simulink model "mrefrobotarm_modified_previous_y_previous_u_previous_ref_pert_2"  (R2018b)
settings: Solver=FixedStepAuto  StartTime=0.0  StopTime=60  RelTol=1e-3  AbsTol=1e-6
undefined symbols (not defined in the file or in its folder): cc, options
libraries: neural x858, simulink x1
(part 8 of 32)

== system mrefrobotarm_modified_previous_y_previous_u_previous_ref_pert_2/m=0 sd=0 new/Layer 3/Delays 1 ==
  "p{3}" : Inport  PortDimensions=30
      mask Display: e = 0.06;c1 = [120 230 180]/255;c2 = ([120 230 180]+0)/(256+128);c3 = ([120 230 180]+128)/(256+128);patch([0 1 1 0],[0 0 1 1],c1);patch([0 1 1 1-e 1-e 0+e],[0 0 1 1-e 0+e 0+e],c2);patch([0 0 1 1-e 0+e 0+e],[0 1 1 1-e 1-e 0+e],c3);plot([0 1 1 0 0],[0 0 1 1 0]);
  mux : Mux  Inputs=1
      mask Display: e = 0.06;c1 = [120 150 230]/255;c2 = ([120 150 230]+0)/383;c3 = ([120 150 230]+128)/383;patch([0 1 1 0],[0 0 1 1],c1);patch([0 1 1 1-e 1-e 0+e],[0 0 1 1-e 0+e 0+e],c2);patch([0 0 1 1-e 0+e 0+e],[0 1 1 1-e 1-e 0+e],c3);plot([0 1 1 0 0],[0 0 1 1 0]);disp('Mux')
  "pd{3,2}" : Outport
      mask Display: e = 0.06;c1 = [120 230 180]/255;c2 = ([120 230 180]+0)/(256+128);c3 = ([120 230 180]+128)/(256+128);patch([0 1 1 0],[0 0 1 1],c1);patch([0 1 1 1-e 1-e 0+e],[0 0 1 1-e 0+e 0+e],c2);patch([0 0 1 1-e 0+e 0+e],[0 1 1 1-e 1-e 0+e],c3);plot([0 1 1 0 0],[0 0 1 1 0]);
  wires:
  "p{3}"/1 -> mux/1
  mux/1 -> "pd{3,2}"/1

== system mrefrobotarm_modified_previous_y_previous_u_previous_ref_pert_2/m=0 sd=0 new/Layer 3/LW{3,2} ==
  "ad{3,2}" : Inport  PortDimensions=30
      mask Display: e = 0.06;c1 = [120 230 180]/255;c2 = ([120 230 180]+0)/(256+128);c3 = ([120 230 180]+128)/(256+128);patch([0 1 1 0],[0 0 1 1],c1);patch([0 1 1 1-e 1-e 0+e],[0 0 1 1-e 0+e 0+e],c2);patch([0 0 1 1-e 0+e 0+e],[0 1 1 1-e 1-e 0+e],c3);plot([0 1 1 0 0],[0 0 1 1 0]);
  "IW{3,2}(1,:)'" : Constant  Value=[-0.131328794563046191701261022899416275322437286376953125;-0.2584338741751863732787342087249271571636199951171875;-0.0903219952940264858565200256634852848947048187255859375;-0.024805674677310464437685055827387259341776371002197265625;0.3313165319494135729883055319078266620635986328125;-0.1756848520066605912059998217955580912530422210693359375;0.62966251824317842622491525617078877985477447509765625;0.002210739002808526608434558369253863929770886898040771484375;0.003937183106850739543192130298621123074553906917572021484375;-0.0763844646287754613922516000457108020782470703125;0.08029708353647936613928237647996866144239902496337890625;-0.059445415608557324038674352095767972059547901153564453125;-0.4850157429702022238160452616284601390361785888671875;-0.1966069396515301159755750859403633512556552886962890625;0.015572684574274832380869071357665234245359897613525390625;0.10249042766198744602856862684348016045987606048583984375;0.259898651756895804343372446965076960623264312744140625;-0.007831826389256744958000666656516841612756252288818359375;-0.060342808177259003865611219907805207185447216033935546875;0.2102990586238534242990994016508921049535274505615234375;-0.054344878005701487133638494242404703982174396514892578125;-0.491551020946996597427158803839120082557201385498046875;-0.57063893253863418042470811997191049158573150634765625;-0.040752953733789419599187198173240176402032375335693359375;0.385146883729147571084894252635422162711620330810546875;-0.49669180336826268540306728027644567191600799560546875;-0.000294463483847452571484648586874754983000457286834716796875;0.402555479876675115225026502230321057140827178955078125;0.0840813874034800623480379044849541969597339630126953125;0.489528113088271099595516488989233039319515228271484375]
      mask Display: e = 0.06;c1 = [120 150 230]/255;c2 = ([120 150 230]+0)/383;c3 = ([120 150 230]+128)/383;patch([0 1 1 0],[0 0 1 1],c1);patch([0 1 1 1-e 1-e 0+e],[0 0 1 1-e 0+e 0+e],c2);patch([0 0 1 1-e 0+e 0+e],[0 1 1 1-e 1-e 0+e],c3);plot([0 1 1 0 0],[0 0 1 1 0]);disp('weights');
  Mux : Mux  Inputs=1
      mask Display: e = 0.06;c1 = [120 150 230]/255;c2 = ([120 150 230]+0)/383;c3 = ([120 150 230]+128)/383;patch([0 1 1 0],[0 0 1 1],c1);patch([0 1 1 1-e 1-e 0+e],[0 0 1 1-e 0+e 0+e],c2);patch([0 0 1 1-e 0+e 0+e],[0 1 1 1-e 1-e 0+e],c3);plot([0 1 1 0 0],[0 0 1 1 0]);disp('Mux');
  dotprod1 : neural/Weight Functions/dotprod
  "lz{3,2}" : Outport
      mask Display: e = 0.06;c1 = [120 230 180]/255;c2 = ([120 230 180]+0)/(256+128);c3 = ([120 230 180]+128)/(256+128);patch([0 1 1 0],[0 0 1 1],c1);patch([0 1 1 1-e 1-e 0+e],[0 0 1 1-e 0+e 0+e],c2);patch([0 0 1 1-e 0+e 0+e],[0 1 1 1-e 1-e 0+e],c3);plot([0 1 1 0 0],[0 0 1 1 0]);
  wires:
  "IW{3,2}(1,:)'"/1 -> dotprod1/1
  "ad{3,2}"/1 -> dotprod1/2
  dotprod1/1 -> Mux/1
  Mux/1 -> "lz{3,2}"/1

== system mrefrobotarm_modified_previous_y_previous_u_previous_ref_pert_2/m=0 sd=0 original/Layer 1/Delays 1 ==
  "p{1}" : Inport  PortDimensions=10
      mask Display: e = 0.06;c1 = [120 230 180]/255;c2 = ([120 230 180]+0)/(256+128);c3 = ([120 230 180]+128)/(256+128);patch([0 1 1 0],[0 0 1 1],c1);patch([0 1 1 1-e 1-e 0+e],[0 0 1 1-e 0+e 0+e],c2);patch([0 0 1 1-e 0+e 0+e],[0 1 1 1-e 1-e 0+e],c3);plot([0 1 1 0 0],[0 0 1 1 0]);
  mux : Mux  Inputs=1
      mask Display: e = 0.06;c1 = [120 150 230]/255;c2 = ([120 150 230]+0)/383;c3 = ([120 150 230]+128)/383;patch([0 1 1 0],[0 0 1 1],c1);patch([0 1 1 1-e 1-e 0+e],[0 0 1 1-e 0+e 0+e],c2);patch([0 0 1 1-e 0+e 0+e],[0 1 1 1-e 1-e 0+e],c3);plot([0 1 1 0 0],[0 0 1 1 0]);disp('Mux')
  "pd{1,1}" : Outport
      mask Display: e = 0.06;c1 = [120 230 180]/255;c2 = ([120 230 180]+0)/(256+128);c3 = ([120 230 180]+128)/(256+128);patch([0 1 1 0],[0 0 1 1],c1);patch([0 1 1 1-e 1-e 0+e],[0 0 1 1-e 0+e 0+e],c2);patch([0 0 1 1-e 0+e 0+e],[0 1 1 1-e 1-e 0+e],c3);plot([0 1 1 0 0],[0 0 1 1 0]);
  wires:
  "p{1}"/1 -> mux/1
  mux/1 -> "pd{1,1}"/1

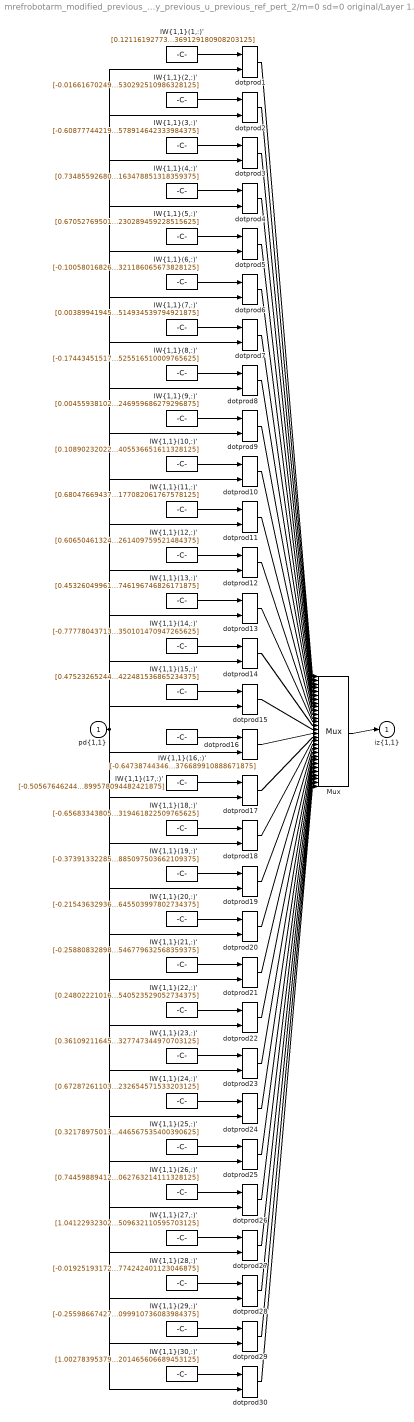
== system mrefrobotarm_modified_previous_y_previous_u_previous_ref_pert_2/m=0 sd=0 original/Layer 1/IW{1,1} ==
  "pd{1,1}" : Inport  PortDimensions=10
      mask Display: e = 0.06;c1 = [120 230 180]/255;c2 = ([120 230 180]+0)/(256+128);c3 = ([120 230 180]+128)/(256+128);patch([0 1 1 0],[0 0 1 1],c1);patch([0 1 1 1-e 1-e 0+e],[0 0 1 1-e 0+e 0+e],c2);patch([0 0 1 1-e 0+e 0+e],[0 1 1 1-e 1-e 0+e],c3);plot([0 1 1 0 0],[0 0 1 1 0]);
  "IW{1,1}(1,:)'" : Constant  Value=[0.12116192773643101598946003605306032113730907440185546875;-0.61504051461735576022960003683692775666713714599609375;0.1409010722643941893039709611912257969379425048828125;0.6780888328524288244381068579968996345996856689453125;1.099852074699011250658031713101081550121307373046875;0.1056636417972652564056801338665536604821681976318359375;-0.12249335544031504652284780831905663944780826568603515625;-1.023192361940513439577671306324191391468048095703125;0.52555112062766362601706759960507042706012725830078125;0.10235940031612085487910945857947808690369129180908203125]
      mask Display: e = 0.06;c1 = [120 150 230]/255;c2 = ([120 150 230]+0)/383;c3 = ([120 150 230]+128)/383;patch([0 1 1 0],[0 0 1 1],c1);patch([0 1 1 1-e 1-e 0+e],[0 0 1 1-e 0+e 0+e],c2);patch([0 0 1 1-e 0+e 0+e],[0 1 1 1-e 1-e 0+e],c3);plot([0 1 1 0 0],[0 0 1 1 0]);disp('Weights');
  "IW{1,1}(10,:)'" : Constant  Value=[0.10890232022583896942524717132982914336025714874267578125;0.65770880199305470359405489944037981331348419189453125;0.457449558769818132031304003248806111514568328857421875;0.78591806431375488273260998539626598358154296875;-0.2188123800257306961203340733845834620296955108642578125;-0.48560017494878715549333492162986658513545989990234375;0.69434633131231038305486436001956462860107421875;-0.328009816819692989753320944146253168582916259765625;0.476343472120701771910233901508036069571971893310546875;0.4472870790745435698454457451589405536651611328125]
      mask Display: e = 0.06;c1 = [120 150 230]/255;c2 = ([120 150 230]+0)/383;c3 = ([120 150 230]+128)/383;patch([0 1 1 0],[0 0 1 1],c1);patch([0 1 1 1-e 1-e 0+e],[0 0 1 1-e 0+e 0+e],c2);patch([0 0 1 1-e 0+e 0+e],[0 1 1 1-e 1-e 0+e],c3);plot([0 1 1 0 0],[0 0 1 1 0]);disp('Weights');
  "IW{1,1}(11,:)'" : Constant  Value=[0.680476694371919155202022011508233845233917236328125;-0.218609157014526156448397387066506780683994293212890625;0.6994701698477083784410979205858893692493438720703125;-0.75912984076269884869958559647784568369388580322265625;-0.053406333734809241509111643608775921165943145751953125;0.5067473596839289218252133650821633636951446533203125;-0.7233312131331359751129639334976673126220703125;0.0220245977869557851835935480266925878822803497314453125;-0.317828864736112548516899778405786491930484771728515625;-0.83728896145760878244601599362795241177082061767578125]
      mask Display: e = 0.06;c1 = [120 150 230]/255;c2 = ([120 150 230]+0)/383;c3 = ([120 150 230]+128)/383;patch([0 1 1 0],[0 0 1 1],c1);patch([0 1 1 1-e 1-e 0+e],[0 0 1 1-e 0+e 0+e],c2);patch([0 0 1 1-e 0+e 0+e],[0 1 1 1-e 1-e 0+e],c3);plot([0 1 1 0 0],[0 0 1 1 0]);disp('Weights');
  "IW{1,1}(12,:)'" : Constant  Value=[0.60650461324363258430736323134624399244785308837890625;0.48153819852384860400462684992817230522632598876953125;-0.04870024737972040995703792987114866264164447784423828125;-0.460239770351729193809120488367625512182712554931640625;-0.368942033692632731511906740706763230264186859130859375;-0.46185690513962518455315375831560231745243072509765625;0.72748634836911574286233417296898551285266876220703125;-0.1586777055629144117521178714014240540564060211181640625;-0.950068089025934536806516916840337216854095458984375;-1.257733091633853828028577481745742261409759521484375]
      mask Display: e = 0.06;c1 = [120 150 230]/255;c2 = ([120 150 230]+0)/383;c3 = ([120 150 230]+128)/383;patch([0 1 1 0],[0 0 1 1],c1);patch([0 1 1 1-e 1-e 0+e],[0 0 1 1-e 0+e 0+e],c2);patch([0 0 1 1-e 0+e 0+e],[0 1 1 1-e 1-e 0+e],c3);plot([0 1 1 0 0],[0 0 1 1 0]);disp('Weights');
  "IW{1,1}(13,:)'" : Constant  Value=[0.4532604996160010113470661963219754397869110107421875;0.09983497416402796476031511474502622149884700775146484375;0.3006063337801030410645353185827843844890594482421875;-0.09180389202883994237414100325622712261974811553955078125;-0.79528576080610113852031872738734818994998931884765625;-0.8960113888966159123583565815351903438568115234375;0.6124459313106982438768000065465457737445831298828125;-0.403120513671325564342140523876878432929515838623046875;0.275852681892310103162202494786470197141170501708984375;-0.9322307026330818313653026052634231746196746826171875]
      mask Display: e = 0.06;c1 = [120 150 230]/255;c2 = ([120 150 230]+0)/383;c3 = ([120 150 230]+128)/383;patch([0 1 1 0],[0 0 1 1],c1);patch([0 1 1 1-e 1-e 0+e],[0 0 1 1-e 0+e 0+e],c2);patch([0 0 1 1-e 0+e 0+e],[0 1 1 1-e 1-e 0+e],c3);plot([0 1 1 0 0],[0 0 1 1 0]);disp('Weights');
  "IW{1,1}(14,:)'" : Constant  Value=[-0.777780437137306268624570293468423187732696533203125;0.54311407500627495448242143538664095103740692138671875;0.1282828683578548789601114776814938522875308990478515625;-0.492876417301822022931645506105269305408000946044921875;0.16977207513145187167680205675424076616764068603515625;0.0156211573477218201855265533595229499042034149169921875;-0.446744619223521599593595965416170656681060791015625;0.75446679844643182999419650514028035104274749755859375;-0.92919935058635305669128001682111062109470367431640625;-0.77293975111376289621745172553346492350101470947265625]
      mask Display: e = 0.06;c1 = [120 150 230]/255;c2 = ([120 150 230]+0)/383;c3 = ([120 150 230]+128)/383;patch([0 1 1 0],[0 0 1 1],c1);patch([0 1 1 1-e 1-e 0+e],[0 0 1 1-e 0+e 0+e],c2);patch([0 0 1 1-e 0+e 0+e],[0 1 1 1-e 1-e 0+e],c3);plot([0 1 1 0 0],[0 0 1 1 0]);disp('Weights');
  "IW{1,1}(15,:)'" : Constant  Value=[0.475232652444419423343191510866745375096797943115234375;-0.96121566108966671748703447519801557064056396484375;-0.57026523941225215619255095589323900640010833740234375;0.377850789131591924263631199210067279636859893798828125;-0.246530389897684221178764119031256996095180511474609375;-0.2456529829883446203186991851907805539667606353759765625;-0.01169546179904616851896737017568739247508347034454345703125;0.04941958440568117172375650625326670706272125244140625;0.2692933235009551395933158346451818943023681640625;-0.98507416687839943758575600440963171422481536865234375]
      mask Display: e = 0.06;c1 = [120 150 230]/255;c2 = ([120 150 230]+0)/383;c3 = ([120 150 230]+128)/383;patch([0 1 1 0],[0 0 1 1],c1);patch([0 1 1 1-e 1-e 0+e],[0 0 1 1-e 0+e 0+e],c2);patch([0 0 1 1-e 0+e 0+e],[0 1 1 1-e 1-e 0+e],c3);plot([0 1 1 0 0],[0 0 1 1 0]);disp('Weights');
  "IW{1,1}(16,:)'" : Constant  Value=[-0.6473874434633859475951567219453863799571990966796875;0.07619240517464466455610505590811953879892826080322265625;0.60985403944523730590532295536831952631473541259765625;0.4716409511471406634797176593565382063388824462890625;-0.9407261485054314587017643134458921849727630615234375;0.469394008329378664701181378404726274311542510986328125;0.86159731456515220582303982155281119048595428466796875;-0.264297224920746531839910176131525076925754547119140625;0.378541128305662055719693626087973825633525848388671875;0.0612841587337953352943031859467737376689910888671875]
      mask Display: e = 0.06;c1 = [120 150 230]/255;c2 = ([120 150 230]+0)/383;c3 = ([120 150 230]+128)/383;patch([0 1 1 0],[0 0 1 1],c1);patch([0 1 1 1-e 1-e 0+e],[0 0 1 1-e 0+e 0+e],c2);patch([0 0 1 1-e 0+e 0+e],[0 1 1 1-e 1-e 0+e],c3);plot([0 1 1 0 0],[0 0 1 1 0]);disp('Weights');
  "IW{1,1}(17,:)'" : Constant  Value=[-0.50567646244606390126818951102904975414276123046875;-0.58678927891174470499180415572482161223888397216796875;-0.74791607997321796208467503674910403788089752197265625;0.09226660376835309207432800349124590866267681121826171875;-0.92881420303231576607316810623160563409328460693359375;0.2054439465067338377313177488758810795843601226806640625;-0.06644508752851059629751517832119134254753589630126953125;-0.0218069911409425921944293946808102191425859928131103515625;-0.4008602233399602976504638718324713408946990966796875;-0.20735309908321475358405905353720299899578094482421875]
      mask Display: e = 0.06;c1 = [120 150 230]/255;c2 = ([120 150 230]+0)/383;c3 = ([120 150 230]+128)/383;patch([0 1 1 0],[0 0 1 1],c1);patch([0 1 1 1-e 1-e 0+e],[0 0 1 1-e 0+e 0+e],c2);patch([0 0 1 1-e 0+e 0+e],[0 1 1 1-e 1-e 0+e],c3);plot([0 1 1 0 0],[0 0 1 1 0]);disp('Weights');
  "IW{1,1}(18,:)'" : Constant  Value=[-0.65683343805488114686141898346249945461750030517578125;0.58491845632951022793122319853864610195159912109375;-0.59386776290678866541128400058369152247905731201171875;0.3328090742596827578125839863787405192852020263671875;-0.40228141483918589127455334164551459252834320068359375;0.56176553124188155496909757857793010771274566650390625;-0.2134990708425597294439768347729113884270191192626953125;0.179285623717090170092802736689918674528598785400390625;0.68978737180453542077174233781988732516765594482421875;0.08143197107304323001386592295602895319461822509765625]
      mask Display: e = 0.06;c1 = [120 150 230]/255;c2 = ([120 150 230]+0)/383;c3 = ([120 150 230]+128)/383;patch([0 1 1 0],[0 0 1 1],c1);patch([0 1 1 1-e 1-e 0+e],[0 0 1 1-e 0+e 0+e],c2);patch([0 0 1 1-e 0+e 0+e],[0 1 1 1-e 1-e 0+e],c3);plot([0 1 1 0 0],[0 0 1 1 0]);disp('Weights');
  "IW{1,1}(19,:)'" : Constant  Value=[-0.37391332285017286896078303470858372747898101806640625;-0.41655114369798862394844718437525443732738494873046875;-0.722962656029874750629460322670638561248779296875;0.74460868870904572958124845172278583049774169921875;0.12195982058353192767352624059640220366418361663818359375;0.573352625586788011702310541295446455478668212890625;-0.6910118607599298190535819230717606842517852783203125;-0.142900412155376133060968868448981083929538726806640625;0.359668576337890122385232416490907780826091766357421875;0.94236811046126600643901838338933885097503662109375]
      mask Display: e = 0.06;c1 = [120 150 230]/255;c2 = ([120 150 230]+0)/383;c3 = ([120 150 230]+128)/383;patch([0 1 1 0],[0 0 1 1],c1);patch([0 1 1 1-e 1-e 0+e],[0 0 1 1-e 0+e 0+e],c2);patch([0 0 1 1-e 0+e 0+e],[0 1 1 1-e 1-e 0+e],c3);plot([0 1 1 0 0],[0 0 1 1 0]);disp('Weights');
  "IW{1,1}(2,:)'" : Constant  Value=[-0.0166167024917292759089715303844059235416352748870849609375;-0.357126463452990094982197888384689576923847198486328125;-0.916084382600150348707757075317203998565673828125;0.48655534141628298261395002555218525230884552001953125;-0.6016239976947996836997845093719661235809326171875;0.2604062173688583836650423108949325978755950927734375;-0.76106782890995205992368255465407855808734893798828125;0.68944498864043690655734053507330827414989471435546875;-0.749670894554280042854088605963625013828277587890625;-0.50522142973601547044637527505983598530292510986328125]
      mask Display: e = 0.06;c1 = [120 150 230]/255;c2 = ([120 150 230]+0)/383;c3 = ([120 150 230]+128)/383;patch([0 1 1 0],[0 0 1 1],c1);patch([0 1 1 1-e 1-e 0+e],[0 0 1 1-e 0+e 0+e],c2);patch([0 0 1 1-e 0+e 0+e],[0 1 1 1-e 1-e 0+e],c3);plot([0 1 1 0 0],[0 0 1 1 0]);disp('Weights');
  "IW{1,1}(20,:)'" : Constant  Value=[-0.2154363293600259077198444401801680214703083038330078125;0.50329604582178533167535761094768531620502471923828125;0.2169027594365723066172080280011869035661220550537109375;-0.1924528806850759055091515392632572911679744720458984375;0.7673985167013552821657640379271470010280609130859375;-0.90934673281269251532421549200080335140228271484375;-0.0087332413715192173941925801727848011068999767303466796875;-0.06668438227395256934215694855083711445331573486328125;-0.016986997923331130511126474402772146277129650115966796875;-0.53458303631503178987571800462319515645503997802734375]
      mask Display: e = 0.06;c1 = [120 150 230]/255;c2 = ([120 150 230]+0)/383;c3 = ([120 150 230]+128)/383;patch([0 1 1 0],[0 0 1 1],c1);patch([0 1 1 1-e 1-e 0+e],[0 0 1 1-e 0+e 0+e],c2);patch([0 0 1 1-e 0+e 0+e],[0 1 1 1-e 1-e 0+e],c3);plot([0 1 1 0 0],[0 0 1 1 0]);disp('Weights');
  "IW{1,1}(21,:)'" : Constant  Value=[-0.258808328980351609605037310757325030863285064697265625;-0.45559647879383280422160851230728439986705780029296875;0.93620596257909582948997240237076766788959503173828125;-0.142913494694684839458886926877312362194061279296875;-0.6309221664067627965977180792833678424358367919921875;0.09462987497119475233109398004671675153076648712158203125;-0.196676609376249034166761475717066787183284759521484375;0.340897810232632381133299759312649257481098175048828125;-0.60326966103195489576904719797312282025814056396484375;-0.1614198301976775551391796170719317160546779632568359375]
      mask Display: e = 0.06;c1 = [120 150 230]/255;c2 = ([120 150 230]+0)/383;c3 = ([120 150 230]+128)/383;patch([0 1 1 0],[0 0 1 1],c1);patch([0 1 1 1-e 1-e 0+e],[0 0 1 1-e 0+e 0+e],c2);patch([0 0 1 1-e 0+e 0+e],[0 1 1 1-e 1-e 0+e],c3);plot([0 1 1 0 0],[0 0 1 1 0]);disp('Weights');
  "IW{1,1}(22,:)'" : Constant  Value=[0.2480222101606265050488531187511398456990718841552734375;0.09883537976841751115930634341566474176943302154541015625;-0.54001494512905789946444201632402837276458740234375;-0.526715938672090100425293712760321795940399169921875;0.58119636565368903990957960559171624481678009033203125;0.37277994148824034059686027831048704683780670166015625;0.5963367799875081143312627318664453923702239990234375;0.0065429653912110440072691375235081068240106105804443359375;-0.73075576347838533397549554138095118105411529541015625;0.6130343513817047007563587612821720540523529052734375]
      mask Display: e = 0.06;c1 = [120 150 230]/255;c2 = ([120 150 230]+0)/383;c3 = ([120 150 230]+128)/383;patch([0 1 1 0],[0 0 1 1],c1);patch([0 1 1 1-e 1-e 0+e],[0 0 1 1-e 0+e 0+e],c2);patch([0 0 1 1-e 0+e 0+e],[0 1 1 1-e 1-e 0+e],c3);plot([0 1 1 0 0],[0 0 1 1 0]);disp('Weights');
  "IW{1,1}(23,:)'" : Constant  Value=[0.36109211645897498765833688594284467399120330810546875;0.54290639213263347517823831367422826588153839111328125;0.07594005242914191045056071516228257678449153900146484375;-0.2461072773103850364062594735514721833169460296630859375;-0.83697661529656885992523029926815070211887359619140625;0.9408581410656988719409810073557309806346893310546875;-0.468248142498214947604395774760632775723934173583984375;-0.2143536848566931218851294715932453982532024383544921875;0.3274754933856305338935044346726499497890472412109375;-0.132677823786770343605923017094028182327747344970703125]
      mask Display: e = 0.06;c1 = [120 150 230]/255;c2 = ([120 150 230]+0)/383;c3 = ([120 150 230]+128)/383;patch([0 1 1 0],[0 0 1 1],c1);patch([0 1 1 1-e 1-e 0+e],[0 0 1 1-e 0+e 0+e],c2);patch([0 0 1 1-e 0+e 0+e],[0 1 1 1-e 1-e 0+e],c3);plot([0 1 1 0 0],[0 0 1 1 0]);disp('Weights');
  "IW{1,1}(24,:)'" : Constant  Value=[0.6728726110333596022172741868416778743267059326171875;-0.8539407689115485755593226713244803249835968017578125;0.58299054175247189135689040995202958583831787109375;0.5965624611944964073018127237446606159210205078125;0.6125643432399214827199784849653951823711395263671875;-0.63478040904533561405997943438705988228321075439453125;-0.32505227239285205964591796146123670041561126708984375;-0.333898527368930275738279078723280690610408782958984375;0.47305369145102804662172957250731997191905975341796875;-0.5194015100786106842178924125619232654571533203125]
      mask Display: e = 0.06;c1 = [120 150 230]/255;c2 = ([120 150 230]+0)/383;c3 = ([120 150 230]+128)/383;patch([0 1 1 0],[0 0 1 1],c1);patch([0 1 1 1-e 1-e 0+e],[0 0 1 1-e 0+e 0+e],c2);patch([0 0 1 1-e 0+e 0+e],[0 1 1 1-e 1-e 0+e],c3);plot([0 1 1 0 0],[0 0 1 1 0]);disp('Weights');
  "IW{1,1}(25,:)'" : Constant  Value=[0.321789750139932217987137619275017641484737396240234375;-0.91569031640294495932863583220751024782657623291015625;-0.333761809396514841363767800430650822818279266357421875;0.7720546237362537755899438707274384796619415283203125;0.51198543788465411541466210110229440033435821533203125;0.824723342100778467056443332694470882415771484375;-0.33046471004821231787218493991531431674957275390625;-0.389875021002500543598756621577194891870021820068359375;0.5404086892708424016973367542959749698638916015625;0.330923257377163049230972546865814365446567535400390625]
      mask Display: e = 0.06;c1 = [120 150 230]/255;c2 = ([120 150 230]+0)/383;c3 = ([120 150 230]+128)/383;patch([0 1 1 0],[0 0 1 1],c1);patch([0 1 1 1-e 1-e 0+e],[0 0 1 1-e 0+e 0+e],c2);patch([0 0 1 1-e 0+e 0+e],[0 1 1 1-e 1-e 0+e],c3);plot([0 1 1 0 0],[0 0 1 1 0]);disp('Weights');
  "IW{1,1}(26,:)'" : Constant  Value=[0.74459889412126256669210988548002205789089202880859375;-0.92984896899672364600775154030998237431049346923828125;0.37858439602939097934353185337386094033718109130859375;-0.198109382923818466704091179053648374974727630615234375;0.8930802272104247929718212617444805800914764404296875;-0.08305259436108174131430104125684010796248912811279296875;0.2584402796521445555555374085088260471820831298828125;-0.1276313566322919423878801126193138770759105682373046875;0.129711283535910160136239710482186637818813323974609375;0.8884779581083848132294633614947088062763214111328125]
      mask Display: e = 0.06;c1 = [120 150 230]/255;c2 = ([120 150 230]+0)/383;c3 = ([120 150 230]+128)/383;patch([0 1 1 0],[0 0 1 1],c1);patch([0 1 1 1-e 1-e 0+e],[0 0 1 1-e 0+e 0+e],c2);patch([0 0 1 1-e 0+e 0+e],[0 1 1 1-e 1-e 0+e],c3);plot([0 1 1 0 0],[0 0 1 1 0]);disp('Weights');
  "IW{1,1}(27,:)'" : Constant  Value=[1.0412293230277336331113247069879435002803802490234375;0.378240268704322979420595629562740214169025421142578125;0.07225563123705869283952551995753310620784759521484375;-0.84672746672924736888177221771911717951297760009765625;-0.92490468420280269601363443143782205879688262939453125;0.22823534262087463719836932796170003712177276611328125;-0.73329745087433939598753340760595165193080902099609375;0.1683653579491500018594507537272875197231769561767578125;-0.017424600058409463188002774813867290504276752471923828125;-0.341270477338222744112528062032652087509632110595703125]
      mask Display: e = 0.06;c1 = [120 150 230]/255;c2 = ([120 150 230]+0)/383;c3 = ([120 150 230]+128)/383;patch([0 1 1 0],[0 0 1 1],c1);patch([0 1 1 1-e 1-e 0+e],[0 0 1 1-e 0+e 0+e],c2);patch([0 0 1 1-e 0+e 0+e],[0 1 1 1-e 1-e 0+e],c3);plot([0 1 1 0 0],[0 0 1 1 0]);disp('Weights');
  "IW{1,1}(28,:)'" : Constant  Value=[-0.019251931722092309462457393465228960849344730377197265625;0.335699510860663907774181780041544698178768157958984375;-0.22472946705043839177307063437183387577533721923828125;0.315214660686319703142288517483393661677837371826171875;-0.176498236704149602527280649155727587640285491943359375;0.31912578476095332380424451912404038012027740478515625;1.1358118760290063509188485113554634153842926025390625;0.50415117773524731337175808221218176186084747314453125;0.2886850425787861329496308826492168009281158447265625;0.7670891568288478179482581253978423774242401123046875]
      mask Display: e = 0.06;c1 = [120 150 230]/255;c2 = ([120 150 230]+0)/383;c3 = ([120 150 230]+128)/383;patch([0 1 1 0],[0 0 1 1],c1);patch([0 1 1 1-e 1-e 0+e],[0 0 1 1-e 0+e 0+e],c2);patch([0 0 1 1-e 0+e 0+e],[0 1 1 1-e 1-e 0+e],c3);plot([0 1 1 0 0],[0 0 1 1 0]);disp('Weights');
  "IW{1,1}(29,:)'" : Constant  Value=[-0.2559866742778955650550187783665023744106292724609375;-0.71127991086725816938240996023523621261119842529296875;-0.41043610779858941128850347013212740421295166015625;0.7048722895097139229392269044183194637298583984375;-0.221963796580707306560498182079754769802093505859375;0.5617244972289625604133789238403551280498504638671875;-0.771930415379233014760984588065184652805328369140625;-0.78155030395383284780308486006106249988079071044921875;0.565621064146131669048145340639166533946990966796875;0.413091510285398921809019157080911099910736083984375]
      mask Display: e = 0.06;c1 = [120 150 230]/255;c2 = ([120 150 230]+0)/383;c3 = ([120 150 230]+128)/383;patch([0 1 1 0],[0 0 1 1],c1);patch([0 1 1 1-e 1-e 0+e],[0 0 1 1-e 0+e 0+e],c2);patch([0 0 1 1-e 0+e 0+e],[0 1 1 1-e 1-e 0+e],c3);plot([0 1 1 0 0],[0 0 1 1 0]);disp('Weights');
  "IW{1,1}(3,:)'" : Constant  Value=[-0.608777442190258977205985502223484218120574951171875;0.85799971456095480704107103520072996616363525390625;-0.74962009257192441236128388482029549777507781982421875;0.192139323756343849414207625159178860485553741455078125;-0.414085422551569493077039396666805259883403778076171875;-0.406854972792761060418342822231352329254150390625;0.484699008415858278997490060646669007837772369384765625;0.285487826019434287605491817885194905102252960205078125;0.56545161713676106440829016719362698495388031005859375;0.09239905289283210920725508685791282914578914642333984375]
      mask Display: e = 0.06;c1 = [120 150 230]/255;c2 = ([120 150 230]+0)/383;c3 = ([120 150 230]+128)/383;patch([0 1 1 0],[0 0 1 1],c1);patch([0 1 1 1-e 1-e 0+e],[0 0 1 1-e 0+e 0+e],c2);patch([0 0 1 1-e 0+e 0+e],[0 1 1 1-e 1-e 0+e],c3);plot([0 1 1 0 0],[0 0 1 1 0]);disp('Weights');
  "IW{1,1}(30,:)'" : Constant  Value=[1.0027839537988934015544373323791660368442535400390625;0.349433229052273919279514302616007626056671142578125;0.362556071783007194397896455484442412853240966796875;-0.250092465292030718959637169973575510084629058837890625;-0.69123761895338731164883938618004322052001953125;0.60623428321575023591805120304343290627002716064453125;-0.0997625681266436081795490053991670720279216766357421875;0.67615237979682085711630179503117688000202178955078125;0.271067671262654796837665571729303337633609771728515625;-0.00512115152377713885034626883907549199648201465606689453125]
      mask Display: e = 0.06;c1 = [120 150 230]/255;c2 = ([120 150 230]+0)/383;c3 = ([120 150 230]+128)/383;patch([0 1 1 0],[0 0 1 1],c1);patch([0 1 1 1-e 1-e 0+e],[0 0 1 1-e 0+e 0+e],c2);patch([0 0 1 1-e 0+e 0+e],[0 1 1 1-e 1-e 0+e],c3);plot([0 1 1 0 0],[0 0 1 1 0]);disp('Weights');
  "IW{1,1}(4,:)'" : Constant  Value=[0.734855926809820036993414760218001902103424072265625;-0.389570311948177872007903488338342867791652679443359375;-0.81885738937908192358605674598948098719120025634765625;1.0182410106540238370342876805807463824748992919921875;-0.464000445312876375059119027355336584150791168212890625;0.212478053400078359391756066543166525661945343017578125;-0.200652031357742732797788676180061884224414825439453125;-0.52859242807870743252607326212455518543720245361328125;-0.77201313289327100353176547287148423492908477783203125;-0.239873280292042689865184001973830163478851318359375]
      mask Display: e = 0.06;c1 = [120 150 230]/255;c2 = ([120 150 230]+0)/383;c3 = ([120 150 230]+128)/383;patch([0 1 1 0],[0 0 1 1],c1);patch([0 1 1 1-e 1-e 0+e],[0 0 1 1-e 0+e 0+e],c2);patch([0 0 1 1-e 0+e 0+e],[0 1 1 1-e 1-e 0+e],c3);plot([0 1 1 0 0],[0 0 1 1 0]);disp('Weights');
  "IW{1,1}(5,:)'" : Constant  Value=[0.67052769501434095200664842195692472159862518310546875;-0.2152872761339806040314925894563202746212482452392578125;0.384828281605536004494894086747081018984317779541015625;-0.6757215826549491932695445939316414296627044677734375;-0.327717615916509108497933766557252965867519378662109375;0.944927686673076028256446079467423260211944580078125;0.85313206769565919085351879402878694236278533935546875;0.26416739724157023427864032782963477075099945068359375;0.429525654215454466555712542685796506702899932861328125;0.1272253550685261969110939617166877724230289459228515625]
      mask Display: e = 0.06;c1 = [120 150 230]/255;c2 = ([120 150 230]+0)/383;c3 = ([120 150 230]+128)/383;patch([0 1 1 0],[0 0 1 1],c1);patch([0 1 1 1-e 1-e 0+e],[0 0 1 1-e 0+e 0+e],c2);patch([0 0 1 1-e 0+e 0+e],[0 1 1 1-e 1-e 0+e],c3);plot([0 1 1 0 0],[0 0 1 1 0]);disp('Weights');
  "IW{1,1}(6,:)'" : Constant  Value=[-0.100580168262270841506023089095833711326122283935546875;-0.82821855871360516854196021085954271256923675537109375;-0.8808772026876916516613391650025732815265655517578125;0.252657513681145307060660343267954885959625244140625;-0.2275202493627272726239851863283547572791576385498046875;0.0031599064136631741135652351459839337621815502643585205078125;-0.310595503818927198835808667354285717010498046875;0.26256673153875331738760223743156529963016510009765625;0.1747747259452554491332421093829907476902008056640625;1.07499825327508791161790213664062321186065673828125]
      mask Display: e = 0.06;c1 = [120 150 230]/255;c2 = ([120 150 230]+0)/383;c3 = ([120 150 230]+128)/383;patch([0 1 1 0],[0 0 1 1],c1);patch([0 1 1 1-e 1-e 0+e],[0 0 1 1-e 0+e 0+e],c2);patch([0 0 1 1-e 0+e 0+e],[0 1 1 1-e 1-e 0+e],c3);plot([0 1 1 0 0],[0 0 1 1 0]);disp('Weights');
  "IW{1,1}(7,:)'" : Constant  Value=[0.0038994194597327630318062130498901751707307994365692138671875;0.67040660914633110056826126310625113546848297119140625;-0.6677336897836270157569060756941325962543487548828125;0.681750229707159149938888731412589550018310546875;-0.485568612997461845903757193809724412858486175537109375;0.36692165947515043011861735067213885486125946044921875;0.72294597873417465461187703112955205142498016357421875;0.540634884828998796280075112008489668369293212890625;-0.434902593385109559331880291210836730897426605224609375;0.6714108410792796188815145796979777514934539794921875]
      mask Display: e = 0.06;c1 = [120 150 230]/255;c2 = ([120 150 230]+0)/383;c3 = ([120 150 230]+128)/383;patch([0 1 1 0],[0 0 1 1],c1);patch([0 1 1 1-e 1-e 0+e],[0 0 1 1-e 0+e 0+e],c2);patch([0 0 1 1-e 0+e 0+e],[0 1 1 1-e 1-e 0+e],c3);plot([0 1 1 0 0],[0 0 1 1 0]);disp('Weights');
  "IW{1,1}(8,:)'" : Constant  Value=[-0.1744345151722600240074001476386911235749721527099609375;-0.368943390105170021531222346311551518738269805908203125;-0.4749454777973067809426765961688943207263946533203125;-0.247239983075249802890738237692858092486858367919921875;0.44350679069850296176724668839597143232822418212890625;0.0102347645488580739348005721467416151426732540130615234375;-0.6757733816479476463001674346742220222949981689453125;0.1963547136057247899376676514293649233877658843994140625;-0.90150897032444399226136511060758493840694427490234375;0.7111578829426312697847833987907506525516510009765625]
      mask Display: e = 0.06;c1 = [120 150 230]/255;c2 = ([120 150 230]+0)/383;c3 = ([120 150 230]+128)/383;patch([0 1 1 0],[0 0 1 1],c1);patch([0 1 1 1-e 1-e 0+e],[0 0 1 1-e 0+e 0+e],c2);patch([0 0 1 1-e 0+e 0+e],[0 1 1 1-e 1-e 0+e],c3);plot([0 1 1 0 0],[0 0 1 1 0]);disp('Weights');
  "IW{1,1}(9,:)'" : Constant  Value=[0.00455938102191570139576359821376172476448118686676025390625;-0.31708861445531477674109055442386306822299957275390625;-0.5208088157022745523505591336288489401340484619140625;-0.2438961511069205612134425109616131521761417388916015625;-0.63715103832776998071807383894338272511959075927734375;-0.745227629189292972711200491175986826419830322265625;-0.591068850718129201737838229746557772159576416015625;0.69980425656285538682510605212883092463016510009765625;0.392129580075222694546255297609604895114898681640625;0.69171599388173188316386585938744246959686279296875]
      mask Display: e = 0.06;c1 = [120 150 230]/255;c2 = ([120 150 230]+0)/383;c3 = ([120 150 230]+128)/383;patch([0 1 1 0],[0 0 1 1],c1);patch([0 1 1 1-e 1-e 0+e],[0 0 1 1-e 0+e 0+e],c2);patch([0 0 1 1-e 0+e 0+e],[0 1 1 1-e 1-e 0+e],c3);plot([0 1 1 0 0],[0 0 1 1 0]);disp('Weights');
  Mux : Mux  Inputs=30
      mask Display: e = 0.06;c1 = [120 150 230]/255;c2 = ([120 150 230]+0)/383;c3 = ([120 150 230]+128)/383;patch([0 1 1 0],[0 0 1 1],c1);patch([0 1 1 1-e 1-e 0+e],[0 0 1 1-e 0+e 0+e],c2);patch([0 0 1 1-e 0+e 0+e],[0 1 1 1-e 1-e 0+e],c3);plot([0 1 1 0 0],[0 0 1 1 0]);disp('Mux');
  dotprod{1..30} (30 alike) : neural/Weight Functions/dotprod
  "iz{1,1}" : Outport
      mask Display: e = 0.06;c1 = [120 230 180]/255;c2 = ([120 230 180]+0)/(256+128);c3 = ([120 230 180]+128)/(256+128);patch([0 1 1 0],[0 0 1 1],c1);patch([0 1 1 1-e 1-e 0+e],[0 0 1 1-e 0+e 0+e],c2);patch([0 0 1 1-e 0+e 0+e],[0 1 1 1-e 1-e 0+e],c3);plot([0 1 1 0 0],[0 0 1 1 0]);
  wires:
  "IW{1,1}(1,:)'"/1 -> dotprod1/1
  "pd{1,1}"/1 -> dotprod1/2, dotprod2/2, dotprod3/2, dotprod4/2, dotprod5/2, dotprod6/2, dotprod7/2, dotprod8/2, dotprod9/2, dotprod10/2, dotprod11/2, dotprod12/2, dotprod13/2, dotprod14/2, dotprod15/2, dotprod16/2, dotprod17/2, dotprod18/2, dotprod19/2, dotprod20/2, dotprod21/2, dotprod22/2, dotprod23/2, dotprod24/2, dotprod25/2, dotprod26/2, dotprod27/2, dotprod28/2, dotprod29/2, dotprod30/2
  dotprod1/1 -> Mux/1
  "IW{1,1}(2,:)'"/1 -> dotprod2/1
  dotprod2/1 -> Mux/2
  "IW{1,1}(3,:)'"/1 -> dotprod3/1
  dotprod3/1 -> Mux/3
  "IW{1,1}(4,:)'"/1 -> dotprod4/1
  dotprod4/1 -> Mux/4
  "IW{1,1}(5,:)'"/1 -> dotprod5/1
  dotprod5/1 -> Mux/5
  "IW{1,1}(6,:)'"/1 -> dotprod6/1
  dotprod6/1 -> Mux/6
  "IW{1,1}(7,:)'"/1 -> dotprod7/1
  dotprod7/1 -> Mux/7
  "IW{1,1}(8,:)'"/1 -> dotprod8/1
  dotprod8/1 -> Mux/8
  "IW{1,1}(9,:)'"/1 -> dotprod9/1
  dotprod9/1 -> Mux/9
  "IW{1,1}(10,:)'"/1 -> dotprod10/1
  dotprod10/1 -> Mux/10
  "IW{1,1}(11,:)'"/1 -> dotprod11/1
  dotprod11/1 -> Mux/11
  "IW{1,1}(12,:)'"/1 -> dotprod12/1
  dotprod12/1 -> Mux/12
  "IW{1,1}(13,:)'"/1 -> dotprod13/1
  dotprod13/1 -> Mux/13
  "IW{1,1}(14,:)'"/1 -> dotprod14/1
  dotprod14/1 -> Mux/14
  "IW{1,1}(15,:)'"/1 -> dotprod15/1
  dotprod15/1 -> Mux/15
  "IW{1,1}(16,:)'"/1 -> dotprod16/1
  dotprod16/1 -> Mux/16
  "IW{1,1}(17,:)'"/1 -> dotprod17/1
  dotprod17/1 -> Mux/17
  "IW{1,1}(18,:)'"/1 -> dotprod18/1
  dotprod18/1 -> Mux/18
  "IW{1,1}(19,:)'"/1 -> dotprod19/1
  dotprod19/1 -> Mux/19
  "IW{1,1}(20,:)'"/1 -> dotprod20/1
  dotprod20/1 -> Mux/20
  "IW{1,1}(21,:)'"/1 -> dotprod21/1
  dotprod21/1 -> Mux/21
  "IW{1,1}(22,:)'"/1 -> dotprod22/1
  dotprod22/1 -> Mux/22
  "IW{1,1}(23,:)'"/1 -> dotprod23/1
  dotprod23/1 -> Mux/23
  "IW{1,1}(24,:)'"/1 -> dotprod24/1
  dotprod24/1 -> Mux/24
  "IW{1,1}(25,:)'"/1 -> dotprod25/1
  dotprod25/1 -> Mux/25
  "IW{1,1}(26,:)'"/1 -> dotprod26/1
  dotprod26/1 -> Mux/26
  "IW{1,1}(27,:)'"/1 -> dotprod27/1
  dotprod27/1 -> Mux/27
  "IW{1,1}(28,:)'"/1 -> dotprod28/1
  dotprod28/1 -> Mux/28
  "IW{1,1}(29,:)'"/1 -> dotprod29/1
  dotprod29/1 -> Mux/29
  "IW{1,1}(30,:)'"/1 -> dotprod30/1
  dotprod30/1 -> Mux/30
  Mux/1 -> "iz{1,1}"/1

== system mrefrobotarm_modified_previous_y_previous_u_previous_ref_pert_2/m=0 sd=0 original/Layer 2/Delays 1 ==
  "p{2}" : Inport  PortDimensions=30
      mask Display: e = 0.06;c1 = [120 230 180]/255;c2 = ([120 230 180]+0)/(256+128);c3 = ([120 230 180]+128)/(256+128);patch([0 1 1 0],[0 0 1 1],c1);patch([0 1 1 1-e 1-e 0+e],[0 0 1 1-e 0+e 0+e],c2);patch([0 0 1 1-e 0+e 0+e],[0 1 1 1-e 1-e 0+e],c3);plot([0 1 1 0 0],[0 0 1 1 0]);
  mux : Mux  Inputs=1
      mask Display: e = 0.06;c1 = [120 150 230]/255;c2 = ([120 150 230]+0)/383;c3 = ([120 150 230]+128)/383;patch([0 1 1 0],[0 0 1 1],c1);patch([0 1 1 1-e 1-e 0+e],[0 0 1 1-e 0+e 0+e],c2);patch([0 0 1 1-e 0+e 0+e],[0 1 1 1-e 1-e 0+e],c3);plot([0 1 1 0 0],[0 0 1 1 0]);disp('Mux')
  "pd{2,1}" : Outport
      mask Display: e = 0.06;c1 = [120 230 180]/255;c2 = ([120 230 180]+0)/(256+128);c3 = ([120 230 180]+128)/(256+128);patch([0 1 1 0],[0 0 1 1],c1);patch([0 1 1 1-e 1-e 0+e],[0 0 1 1-e 0+e 0+e],c2);patch([0 0 1 1-e 0+e 0+e],[0 1 1 1-e 1-e 0+e],c3);plot([0 1 1 0 0],[0 0 1 1 0]);
  wires:
  "p{2}"/1 -> mux/1
  mux/1 -> "pd{2,1}"/1
